simulink model "teste_BP_chebyI"  (R2018a)
settings: Solver=VariableStepAuto  StartTime=0.0  StopTime=10.0  RelTol=1e-3
libraries: dspsrcs4 x1
settings Model: Creator=marco  LastModifiedBy=marco

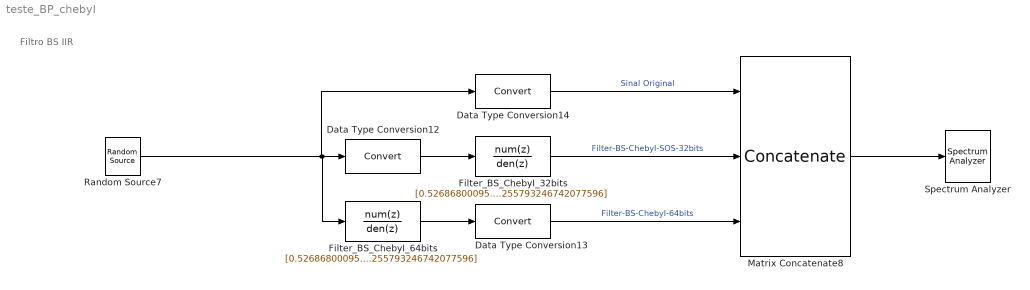
== system teste_BP_chebyI ==
  note: Filtro BS IIR
  Data Type Conversion12 : DataTypeConversion
  Data Type Conversion13 : DataTypeConversion
  Data Type Conversion14 : DataTypeConversion
  Filter_BS_ChebyI_32bits : DiscreteFilter  Tag=BlockMethodSubSystem  Numerator=[0.526868000951233872 -1.54203566956132732 5.62231543277647106 -10.600101182726668 21.298995446777635 -28.6634656336700679 39.4931897641130405 -39.2119772064789842 39.4931897641130405 -28.6634656336700679 21.298995446777635 -10.600101182726668 5.62231543277647106 -1.54203566956132732 0.526868000951233872]  Denominator=[1 -2.66499543662062877 8.79464618040259083 -15.0964799784515531 27.5316314023528577 -33.7583267920149481 42.2783703159670097 -38.2580281440592245 35.0287520822531278 -23.1519310706400248 15.6125822995039183 -7.05648534288835538 3.38096176201517462 -0.836935413720374832 0.255793246742077596]  InputProcessing=Columns as channels (frame based)  a0EqualsOne=on
  Filter_BS_ChebyI_64bits : DiscreteFilter  Tag=BlockMethodSubSystem  Numerator=[0.526868000951233872 -1.54203566956132732 5.62231543277647106 -10.600101182726668 21.298995446777635 -28.6634656336700679 39.4931897641130405 -39.2119772064789842 39.4931897641130405 -28.6634656336700679 21.298995446777635 -10.600101182726668 5.62231543277647106 -1.54203566956132732 0.526868000951233872]  Denominator=[1 -2.66499543662062877 8.79464618040259083 -15.0964799784515531 27.5316314023528577 -33.7583267920149481 42.2783703159670097 -38.2580281440592245 35.0287520822531278 -23.1519310706400248 15.6125822995039183 -7.05648534288835538 3.38096176201517462 -0.836935413720374832 0.255793246742077596]  InputProcessing=Columns as channels (frame based)  a0EqualsOne=on
  Matrix Concatenate8 : Concatenate  NumInputs=3  Mode=Multidimensional array  ConcatenateDimension=2
  Random Source7 : dspsrcs4/Random Source  SrcType=Uniform  NormMethod=Ziggurat  CltLength=12  MinVal=-0.5  MaxVal=0.5  MeanVal=0  VarVal=1  RepMode=Not repeatable  rawSeed=1  IsInherit=off  SampMode=Discrete  SampTime=1/6000  SampFrame=1  DataType=Double  OutComplex=Real  OutputFrames=on
  Spectrum Analyzer : SpectrumAnalyzer
  wires:
  Random Source7/1 -> Data Type Conversion14/1, Data Type Conversion12/1, Filter_BS_ChebyI_64bits/1
  Data Type Conversion13/1 -> Matrix Concatenate8/3  "Filter-BS-ChebyI-64bits"
  Filter_BS_ChebyI_64bits/1 -> Data Type Conversion13/1
  Matrix Concatenate8/1 -> Spectrum Analyzer/1
  Data Type Conversion14/1 -> Matrix Concatenate8/1  "Sinal Original"
  Filter_BS_ChebyI_32bits/1 -> Matrix Concatenate8/2  "Filter-BS-ChebyI-SOS-32bits"
  Data Type Conversion12/1 -> Filter_BS_ChebyI_32bits/1
